simulink model "Stabilizator_cisnienia"  (R2016a)
settings: Solver=VariableStepAuto  StartTime=0.0  StopTime=10.0  RelTol=1e-3
values from neighbouring files (symbols this model uses):
  A_pr = 38.484    [Pressurizer_constants.m]
  AUX0 = 0    [Pressurizer_constants.m]
  AUX_pr0 = 0    [Pressurizer_constants.m]
  G_he = -250    [Pressurizer_constants.m]
  G_he1 = -250    [Pressurizer_constants.m]
  G_sp = 0    [Pressurizer_constants.m]
  G_sp1 = 75    [Pressurizer_constants.m]
  H_fgp0 = 414.8    [Pressurizer_constants.m]
  H_sp = 574.36    [Pressurizer_constants.m]
  H_wi0 = 672.84    [Pressurizer_constants.m]
  H_wp0 = 701.1    [Pressurizer_constants.m]
  J = 5.4027    [Pressurizer_constants.m]
  K_p1 = -0.008152    [Pressurizer_constants.m]
  K_p2 = 0.00470802    [Pressurizer_constants.m]
  K_p3 = 0.118    [Pressurizer_constants.m]
  K_p4 = -0.2081    [Pressurizer_constants.m]
  K_p5 = 5.9e-6    (= 5.9e-06)    [Pressurizer_constants.m]
  K_p6 = -1.118e-4    (= -0.0001118)    [Pressurizer_constants.m]
  K_pr = 0    [Pressurizer_constants.m]
  K_pr1 = 0    [Pressurizer_constants.m]
  L_p = 46.76    [Pressurizer_constants.m]
  L_sp0 = 18.7    [Pressurizer_constants.m]
  L_wp0 = 28.06    [Pressurizer_constants.m]
  M_sp0 = 4588.33    [Pressurizer_constants.m]
  M_wp0 = 40029.65    [Pressurizer_constants.m]
  Pr0 = 2250    [Pressurizer_constants.m]
  Pr1 = 2265    [Pressurizer_constants.m]
  Pr2 = 2275    [Pressurizer_constants.m]
  ro_sp0 = 6.37267    [Pressurizer_constants.m]
  ro_wp0 = 37.064    [Pressurizer_constants.m]
  tau1_pr = 900    [Pressurizer_constants.m]
  tau2_pr = 2    [Pressurizer_constants.m]
  tau3_pr = 200    [Pressurizer_constants.m]
  tau4_pr = 2    [Pressurizer_constants.m]
  V_fp0 = 0.02698    [Pressurizer_constants.m]
  V_gp0 = 0.15692    [Pressurizer_constants.m]
  V_sp0 = 720    [Pressurizer_constants.m]
  V_wp0 = 1080    [Pressurizer_constants.m]
  W_sp = 0    [Pressurizer_constants.m]
  W_sr0 = 0    [Pressurizer_constants.m]
  X_fgp = 883.025    [Pressurizer_constants.m]
  X_fp = 435.6    [Pressurizer_constants.m]
  X_sp = -4.2203    [Pressurizer_constants.m]
  X_vfp = 0.013705    [Pressurizer_constants.m]
  X_vgp = 0.40847    [Pressurizer_constants.m]
  X_wp = 55.406    [Pressurizer_constants.m]
settings Model: Creator=Michal Chruscinski  LastModifiedBy=Michal Chruscinski

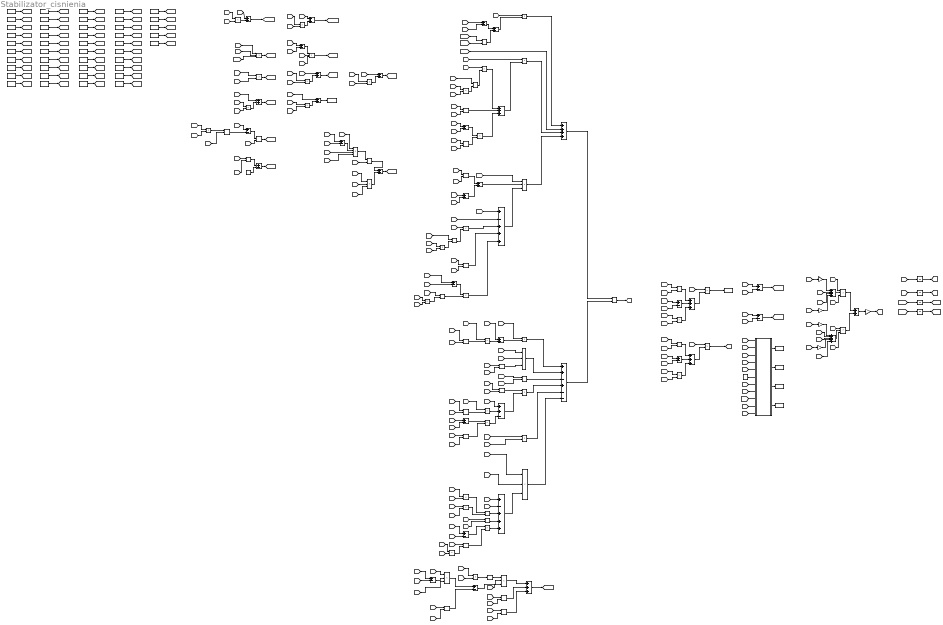
== system Stabilizator_cisnienia ==
  note: INTEGRATION
  note: W_sr
  note: CONTROL SYSTEM
  note: CONTROL PROCEDURE
  note: dAUX
  note: dAUX_pr
  note: dL_wp
  note: EQUATIONS
  note: CONSTANTS
  note: W_sp
  note: dPr
  note: dPr_mianownik
  note: dPr_licznik
  note: Qhe
  AUX0 : Constant  Value=AUX0
  AUX_pr0 : Constant  Value=AUX_pr0
  A_pr : Constant  Value=A_pr
  Add1 : Sum
  Add2 : Sum  Inputs=++++
  Add3 : Sum  Inputs=+++
  Add4 : Sum
  Add5 : Sum
  Apr*(Lp-Lwp)*Kp2 : Product  Inputs=3
  Apr*(Lp-Lwp)*Kp2*ROUwp/ROUsp1 : Product  Inputs=*/
  Apr*(Lp-Lwp)*Kp2*ROUwp1 : Product  Inputs=4
  Apr*Lwp*Kp2 : Product  Inputs=3
  C1p : Sum  Inputs=+-
  C2p/C1p : Product  Inputs=*/
  C2p1 : Sum
  Constant : Constant  Value=K_pr1
  DLwp : Sum  Inputs=+++
  DLwp_drugi_nawias : Sum  Inputs=+-
  DLwp_glowny_iloczyn : Product  Inputs=3
  Divide{1..20} (20 alike) : Product  Inputs=*/
  G_he : Constant  Value=G_he
  G_he1 : Constant  Value=G_he1
  G_sp : Constant  Value=G_sp
  G_sp1 : Constant  Value=G_sp1
  Gain : Gain  Gain=-1
  Gain1 : Gain  Gain=2
  Gain2 : Gain  Gain=1/2
  Gain3 : Gain  Gain=2
  Gain4 : Gain  Gain=1/2
  H_fgp0 : Constant  Value=H_fgp0
  H_fsr : Sum
  H_sp : Constant  Value=H_sp
  H_wi0 : Constant  Value=H_wi0
  H_wp0 : Constant  Value=H_wp0
  Hfsr : Sum
  Integrator : Integrator  InitialCondition=L_wp0
  Integrator1 : Integrator  InitialCondition=Pr0
  Integrator2 : Integrator  InitialCondition=AUX_pr0
  Integrator3 : Integrator  InitialCondition=AUX0
  J : Constant  Value=J
  K_p1 : Constant  Value=K_p1
  K_p2 : Constant  Value=K_p2
  K_p3 : Constant  Value=K_p3
  K_p4 : Constant  Value=K_p4
  K_p5 : Constant  Value=K_p5
  K_p6 : Constant  Value=K_p6
  K_pr : Constant  Value=K_pr
  Kp1 - ROUwp*Kp2/ROUsp : Sum  Inputs=+-
  Kp1*Pr : Product
  Kp2*Pr : Product
  Kp3 * Pr : Product
  Kp4 * Pr : Product
  Kp5 * Pr : Product
  Kp5 * Pr2 : Product
  Kp7 : Product  Inputs=*/
  L_p : Constant  Value=L_p
  L_sp0 : Constant  Value=L_sp0
  L_wp0 : Constant  Value=L_wp0
  Liczba_1 : Constant
  Lp-Lwp : Sum  Inputs=+-
  Lp-Lwp1 : Sum  Inputs=+-
  Lp-Lwp2 : Sum  Inputs=+-
  MATLAB Function : MATLAB Function  TreatAsAtomicUnit=on
  M_sp0 : Constant  Value=M_sp0
  M_wp0 : Constant  Value=M_wp0
  Math Function : Math  Operator=reciprocal  SaturateOnIntegerOverflow=on
  Msp : Product  Inputs=3
  Mwp : Product  Inputs=3
  Pr0 : Constant  Value=Pr0
  Pr1 : Constant  Value=Pr1
  Pr2 : Constant  Value=Pr2
  Product{,1..5,7..11,13..16,18..25} (23 alike) : Product
  Product{6,12,17,26..27} (5 alike) : Product  Inputs=3
  ROUsp : Sum
  ROUsp*Apr : Product
  ROUwp : Sum
  ROUwp*Kp2 : Product
  ROUwp*Kp2/ROUsp : Product  Inputs=*/
  ROUwp/ROUsp : Product  Inputs=*/
  Sub{1..3,5,8,10,12,14..16} (10 alike) : Sum  Inputs=+-
  Sub11 : Sum  Inputs=+++
  Sub13 : Sum  Inputs=+++
  Sub17 : Sum
  Sub18 : Sum  Inputs=++++
  Sub19 : Sum  Inputs=+++++
  Sub4 : Sum  Inputs=+-+++
  Sub6 : Sum  Inputs=++-+--
  Sub7 : Sum  Inputs=++-
  Sub9 : Sum  Inputs=+-+++
  To Workspace : ToWorkspace  VariableName=K_pr1  SaveFormat=Timeseries  SampleTime=-1
  To Workspace1 : ToWorkspace  VariableName=K_pr  SaveFormat=Timeseries  SampleTime=-1
  To Workspace2 : ToWorkspace  VariableName=G_sp  SaveFormat=Timeseries  SampleTime=-1
  To Workspace3 : ToWorkspace  VariableName=G_he  SaveFormat=Timeseries  SampleTime=-1
  To Workspace4 : ToWorkspace  VariableName=W_sp  SaveFormat=Timeseries  SampleTime=-1
  To Workspace5 : ToWorkspace  VariableName=H_fsr  SaveFormat=Timeseries  SampleTime=-1
  V_fp0 : Constant  Value=V_fp0
  V_gp0 : Constant  Value=V_gp0
  V_sp0 : Constant  Value=V_sp0
  V_wp0 : Constant  Value=V_wp0
  Vfp : Sum
  Vfp1 : Sum
  Vwp : Product
  W_sp : Constant  Value=W_sp
  W_sr0 : Constant  Value=W_sr0
  Wsp/C1p : Product  Inputs=*/
  Wsr/C1p1 : Product  Inputs=*/
  X_fgp : Constant  Value=X_fgp
  X_fp : Constant  Value=X_fp
  X_sp : Constant  Value=X_sp
  X_vfp : Constant  Value=X_vfp
  X_vgp : Constant  Value=X_vgp
  X_wp : Constant  Value=X_wp
  ro_sp0 : Constant  Value=ro_sp0
  ro_wp0 : Constant  Value=ro_wp0
  tau1_pr : Constant  Value=tau1_pr
  tau2_pr : Constant  Value=tau2_pr
  tau3_pr : Constant  Value=tau3_pr
  tau4_pr : Constant  Value=tau4_pr
  wires:
  Kp2*Pr/1 -> ROUsp/2
  [X_sp] -> ROUsp/1
  [K_p2] -> Kp2*Pr/1
  Kp1*Pr/1 -> ROUwp/2
  [K_p1] -> Kp1*Pr/1
  DLwp/1 -> [dL_wp]
  ROUwp/1 -> [ro_wp]
  ROUsp/1 -> [ro_sp]
  Kp4 * Pr/1 -> Hfsr/2
  [X_fgp] -> Hfsr/1
  [K_p4] -> Kp4 * Pr/1
  Kp3 * Pr/1 -> H_fsr/2
  [K_p3] -> Kp3 * Pr/1
  [X_fp] -> H_fsr/1
  [X_vfp] -> Vfp/1
  Kp5 * Pr/1 -> Vfp/2
  ROUwp*Kp2/1 -> ROUwp*Kp2/ROUsp/1
  ROUwp*Kp2/ROUsp/1 -> Kp1 - ROUwp*Kp2/ROUsp/2
  Kp1 - ROUwp*Kp2/ROUsp/1 -> Kp7/1
  ROUwp/ROUsp/1 -> C1p/1
  Liczba_1/1 -> C1p/2
  ROUsp*Apr/1 -> Math Function/1
  Math Function/1 -> DLwp_glowny_iloczyn/1
  Apr*(Lp-Lwp)*Kp2/1 -> DLwp_drugi_nawias/1
  C2p/C1p/1 -> DLwp_drugi_nawias/2
  DLwp_drugi_nawias/1 -> DLwp_glowny_iloczyn/2
  Divide9/1 -> [dPr]
  DLwp_glowny_iloczyn/1 -> DLwp/1
  C1p/1 -> [C1_p]
  [W_sp] -> Wsp/C1p/1
  Wsp/C1p/1 -> DLwp/3
  Wsr/C1p1/1 -> DLwp/2
  Mwp/1 -> [M_wp]
  Msp/1 -> [M_sp]
  Vwp/1 -> [V_wp]
  Hfsr/1 -> To Workspace5/1
  H_fsr/1 -> [H_fsr]
  Vfp/1 -> [V_fp]
  Kp7/1 -> [K_p7]
  Sub1/1 -> Add1/1
  Add1/1 -> Product/2
  [Pr0] -> Sub1/2
  [Pr] -> Sub1/1
  Product/1 -> Add2/1
  [K_pr] -> Add2/2
  [W_sr] -> Product1/1
  [C1_p] -> Product3/1
  Product3/1 -> Divide1/2
  [V_fp] -> Divide1/1
  Divide1/1 -> Product2/2
  [Pr] -> Product2/1
  Divide2/1 -> Add1/2
  [tau1_pr] -> Divide2/2
  [AUX_pr] -> Divide2/1
  [H_fgp] -> Divide3/1
  [C1_p] -> Divide3/2
  Divide3/1 -> Add3/2
  Product2/1 -> Add3/1
  Sub2/1 -> Product4/1
  Divide4/1 -> Product4/2
  [V_gp] -> Sub2/1
  [V_fp] -> Sub2/2
  [Pr] -> Divide4/1
  [C1_p] -> Divide4/2
  Product4/1 -> Add3/3
  Add3/1 -> Product1/2
  Product1/1 -> Add2/3
  Add4/1 -> Product6/2
  [AUX] -> Divide5/1
  [tau3_pr] -> Divide5/2
  Divide5/1 -> Add4/1
  [Pr0] -> Sub3/2
  [Pr] -> Sub3/1
  Sub3/1 -> Add4/2
  Sub4/1 -> Product6/3
  [H_fsr] -> Sub4/2
  Divide6/1 -> Product7/2
  Product7/1 -> Sub4/3
  [Pr] -> Product7/1
  Product8/1 -> Divide6/2
  [C1_p] -> Product8/1
  [J] -> Product3/2
  [J] -> Product8/2
  [V_gp] -> Divide6/1
  [H_fgp] -> Divide7/1
  [C1_p] -> Divide7/2
  Divide7/1 -> Sub4/4
  Product9/1 -> Sub4/5
  Sub5/1 -> Product9/1
  [C1_p] -> Product10/1
  [J] -> Product10/2
  Divide8/1 -> Product9/2
  Product10/1 -> Divide8/2
  [Pr] -> Divide8/1
  [V_gp] -> Sub5/1
  [V_fp] -> Sub5/2
  Product6/1 -> Add2/4
  Add2/1 -> Divide9/1
  Sub6/1 -> Divide9/2
  Product5/1 -> Sub6/1
  Add5/1 -> Product5/2
  Product11/1 -> Add5/2
  Divide10/1 -> Product11/2
  [M_wp] -> Product5/1
  [Pr] -> Divide10/1
  [J] -> Divide10/2
  [Pr] -> Divide11/1
  [J] -> Divide11/2
  Product12/1 -> Sub6/2
  [M_sp] -> Product12/1
  [K_p6] -> Product12/2
  Divide11/1 -> Product12/3
  Divide12/1 -> Sub6/3
  [J] -> Divide12/2
  [V_wp] -> Divide12/1
  Product13/1 -> Sub6/4
  Divide13/1 -> Product13/1
  [C1_p] -> Divide13/1
  [C2_p] -> Divide13/2
  Sub7/1 -> Product13/2
  [H_fgp] -> Sub7/1
  Product14/1 -> Sub7/2
  Divide14/1 -> Product14/2
  [J] -> Divide14/2
  [V_fp] -> Divide14/1
  [Pr] -> Product14/1
  Product15/1 -> Sub7/3
  Sub8/1 -> Product15/1
  Divide15/1 -> Product15/2
  [V_fp] -> Sub8/1
  [V_gp] -> Sub8/2
  [Pr] -> Divide15/1
  [J] -> Divide15/2
  Product16/1 -> Sub6/5
  [G_sp] -> Product6/1
  [G_he] -> Product/1
  [G_he] -> Product16/1
  [tau2_pr] -> Product16/2
  Product17/1 -> Sub6/6
  [G_sp] -> Product17/1
  [tau4_pr] -> Product17/2
  Sub9/1 -> Product17/3
  [H_sp] -> Sub4/1
  [H_sp] -> Sub9/1
  [H_fsr] -> Sub9/2
  Divide16/1 -> Sub9/3
  Product19/1 -> Divide16/1
  Product18/1 -> Divide16/2
  [Pr] -> Product19/1
  [V_gp] -> Product19/2
  [C1_p] -> Product18/1
  [J] -> Product18/2
  Divide17/1 -> Sub9/4
  [H_fgp] -> Divide17/1
  [C1_p] -> Divide17/2
  Product20/1 -> Sub9/5
  Divide18/1 -> Product20/2
  Sub10/1 -> Product20/1
  Product21/1 -> Divide18/2
  [V_gp] -> Sub10/1
  [V_fp] -> Sub10/2
  [C1_p] -> Product21/1
  [J] -> Product21/2
  [G_sp] -> Product22/1
  Sub11/1 -> Product22/2
  Divide19/1 -> Sub11/1
  [AUX] -> Divide19/1
  [tau3_pr] -> Divide19/2
  Sub12/1 -> Sub11/2
  [Pr] -> Sub12/1
  [Pr0] -> Sub12/2
  Product23/1 -> Sub11/3
  [tau4_pr] -> Product23/1
  [dPr] -> Product23/2
  Product22/1 -> To Workspace4/1
  [G_he] -> Product24/1
  Sub13/1 -> Product24/2
  Divide20/1 -> Sub13/1
  [AUX_pr] -> Divide20/1
  [tau1_pr] -> Divide20/2
  Sub14/1 -> Sub13/2
  [Pr] -> Sub14/1
  [Pr0] -> Sub14/2
  Product25/1 -> Sub13/3
  [tau2_pr] -> Product25/1
  [dPr] -> Product25/2
  Product24/1 -> [Q_he]
  [Pr] -> Sub15/1
  [Pr0] -> Sub15/2
  [Pr] -> Sub16/1
  [Pr0] -> Sub16/2
  Sub15/1 -> [dAUX_pr]
  Sub16/1 -> [dAUX]
  Constant/1 -> MATLAB Function/6("K_pr1 ")
  MATLAB Function/4(K_pr1) -> To Workspace/1
  [Pr] -> MATLAB Function/2(Pr)
  A_pr/1 -> [A_pr]
  L_wp0/1 -> [L_wp0]
  L_sp0/1 -> [L_sp0]
  V_sp0/1 -> [V_sp0]
  V_wp0/1 -> [V_wp0]
  M_wp0/1 -> [M_wp0]
  M_sp0/1 -> [M_sp0]
  L_p/1 -> [L_p]
  Pr0/1 -> [Pr0]
  H_wp0/1 -> [H_wp0]
  K_p4/1 -> [K_p4]
  K_p5/1 -> [K_p5]
  K_p6/1 -> [K_p6]
  X_wp/1 -> [X_wp]
  X_sp/1 -> [X_sp]
  X_fp/1 -> [X_fp]
  X_fgp/1 -> [X_fgp]
  X_vfp/1 -> [X_vfp]
  X_vgp/1 -> [X_vgp]
  J/1 -> [J]
  W_sr0/1 -> [W_sr0]
  W_sp/1 -> [W_sp]
  G_he/1 -> [G_he]
  G_he1/1 -> [G_he1]
  tau1_pr/1 -> [tau1_pr]
  tau2_pr/1 -> [tau2_pr]
  AUX_pr0/1 -> [AUX_pr0]
  G_sp/1 -> [G_sp]
  G_sp1/1 -> [G_sp1]
  tau3_pr/1 -> [tau3_pr]
  [Pr] -> Kp2*Pr/2
  [X_wp] -> ROUwp/1
  [Pr] -> Kp1*Pr/2
  [A_pr] -> Mwp/2
  [L_wp] -> Mwp/1
  [ro_wp] -> Mwp/3
  [L_p] -> Lp-Lwp/1
  [L_wp] -> Lp-Lwp/2
  [A_pr] -> Msp/2
  [ro_sp] -> Msp/3
  Lp-Lwp/1 -> Msp/1
  [L_wp] -> Vwp/1
  [A_pr] -> Vwp/2
  [Pr] -> Kp3 * Pr/2
  [Pr] -> Kp4 * Pr/2
  [K_p5] -> Kp5 * Pr/1
  [Pr] -> Kp5 * Pr/2
  [X_vgp] -> Vfp1/1
  Kp5 * Pr2/1 -> Vfp1/2
  Vfp1/1 -> [V_gp]
  [K_p6] -> Kp5 * Pr2/1
  [Pr] -> Kp5 * Pr2/2
  [ro_sp] -> Kp7/2
  [K_p1] -> Kp1 - ROUwp*Kp2/ROUsp/1
  [ro_wp] -> ROUwp*Kp2/1
  [K_p2] -> ROUwp*Kp2/2
  [ro_sp] -> ROUwp*Kp2/ROUsp/2
  [ro_sp] -> ROUwp/ROUsp/2
  [ro_wp] -> ROUwp/ROUsp/1
  Apr*(Lp-Lwp)*Kp2*ROUwp1/1 -> Apr*(Lp-Lwp)*Kp2*ROUwp/ROUsp1/1
  Apr*(Lp-Lwp)*Kp2*ROUwp/ROUsp1/1 -> C2p1/1
  Apr*Lwp*Kp2/1 -> C2p1/2
  C2p1/1 -> [C2_p]
  [K_p1] -> Apr*Lwp*Kp2/3
  [A_pr] -> Apr*Lwp*Kp2/1
  [L_wp] -> Apr*Lwp*Kp2/2
  [A_pr] -> Apr*(Lp-Lwp)*Kp2*ROUwp1/1
  [L_p] -> Lp-Lwp1/1
  [L_wp] -> Lp-Lwp1/2
  Lp-Lwp1/1 -> Apr*(Lp-Lwp)*Kp2*ROUwp1/2
  [K_p2] -> Apr*(Lp-Lwp)*Kp2*ROUwp1/3
  [ro_wp] -> Apr*(Lp-Lwp)*Kp2*ROUwp1/4
  [ro_sp] -> Apr*(Lp-Lwp)*Kp2*ROUwp/ROUsp1/2
  [A_pr] -> ROUsp*Apr/1
  [ro_sp] -> ROUsp*Apr/2
  [C1_p] -> Wsp/C1p/2
  [C1_p] -> C2p/C1p/2
  [C2_p] -> C2p/C1p/1
  [dPr] -> DLwp_glowny_iloczyn/3
  [A_pr] -> Apr*(Lp-Lwp)*Kp2/1
  Lp-Lwp2/1 -> Apr*(Lp-Lwp)*Kp2/2
  [L_wp] -> Lp-Lwp2/2
  [L_p] -> Lp-Lwp2/1
  [K_p2] -> Apr*(Lp-Lwp)*Kp2/3
  [W_sr] -> Wsr/C1p1/1
  [C1_p] -> Wsr/C1p1/2
  MATLAB Function/3(K_pr) -> To Workspace1/1
  MATLAB Function/2(G_sp) -> To Workspace2/1
  MATLAB Function/1(G_he) -> To Workspace3/1
  Sub17/1 -> Gain/1
  Product26/1 -> Sub17/1
  Gain/1 -> [W_sr]
  Product27/1 -> Sub17/2
  [B_cl] -> Product26/1
  [B_hl] -> Product27/1
  Sub18/1 -> Product26/2
  Gain1/1 -> Sub18/1
  [V_p] -> Gain1/1
  [V_cl] -> Sub18/2
  [V_lp] -> Sub18/3
  [V_mo] -> Gain2/1
  Gain2/1 -> Sub18/4
  [dT_cl] -> Product26/3
  Gain3/1 -> Sub19/1
  [V_p] -> Gain3/1
  [V_hl] -> Sub19/2
  [V_up] -> Sub19/3
  [V_mo] -> Gain4/1
  Gain4/1 -> Sub19/4
  Sub19/1 -> Product27/2
  [dT_hl] -> Product27/3
  [V_wp0] -> Sub19/5
  Integrator/1 -> [L_wp]
  [dL_wp] -> Integrator/1
  Integrator1/1 -> [Pr]
  [dPr] -> Integrator1/1
  Integrator2/1 -> [AUX_pr]
  [dAUX_pr] -> Integrator2/1
  Integrator3/1 -> [AUX]
  [dAUX] -> Integrator3/1
  [K_p5] -> Product11/1
  [K_p3] -> Add5/1
  K_p3/1 -> [K_p3]
  K_p2/1 -> [K_p2]
  K_p1/1 -> [K_p1]
  V_gp0/1 -> [V_gp0]
  V_fp0/1 -> [V_fp0]
  ro_sp0/1 -> [ro_sp0]
  ro_wp0/1 -> [ro_wp0]
  H_wi0/1 -> [H_wi0]
  H_sp/1 -> [H_sp]
  H_fgp0/1 -> [H_fgp0]
  tau4_pr/1 -> [tau4_pr]
  AUX0/1 -> [AUX0]
  K_pr/1 -> [K_pr]
  Pr1/1 -> [Pr1]
  Pr2/1 -> [Pr2]
  [Pr] -> Divide18/1
  [Pr1] -> MATLAB Function/4(Pr1)
  [Pr2] -> MATLAB Function/5(Pr2)
  [dPr] -> MATLAB Function/1(dPr)
  [Pr0] -> MATLAB Function/3(Pr0)
  [G_he1] -> MATLAB Function/7(G_he1)
  [AUX_pr] -> MATLAB Function/9(AUX_pr)
  [tau1_pr] -> MATLAB Function/10(tau1_pr)
  [tau2_pr] -> MATLAB Function/11(tau2_pr)
  [G_sp1] -> MATLAB Function/8(G_sp1)

== matlab function Stabilizator_cisnienia/MATLAB Function ==
  data: dPr input; Pr input; Pr0 input; Pr1 input; Pr2 input; G_he output; G_sp output; K_pr output; K_pr1 output; K_pr1 input; G_he1 input; G_sp1 input; AUX_pr input; tau1_pr input; tau2_pr input
function [G_he,G_sp,K_pr,K_pr1] = fcn(dPr,Pr,Pr0,Pr1,Pr2,K_pr1,G_he1,G_sp1,AUX_pr,tau1_pr,tau2_pr)
G_he=-250
G_sp=0
K_pr=0
if(Pr<Pr1)
    G_he=-250
    G_sp=0
    K_pr=0
end
if(Pr >= Pr1)
   if(Pr >= Pr2)
       K_pr=K_pr1
       G_he=0
       G_sp=G_sp1
   else
       K_pr1=G_he1*(AUX_pr/tau1_pr+(Pr-Pr0)+tau2_pr*dPr)
       K_pr=K_pr1
       G_he=0
       G_sp=0
   end
end
G_sp2=0
